simulink model "MRACinSimulink"  (R2025b)
settings: Solver=FixedStepAuto  StartTime=0.0  StopTime=100  FixedStep=0.1  RelTol=1e-3
settings Model: Creator=Asus  LastModifiedBy=Asus

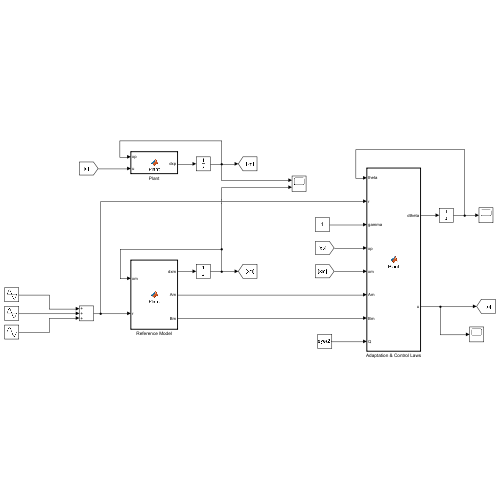
[thumbnail: Simulink's stored preview of the top-level diagram]
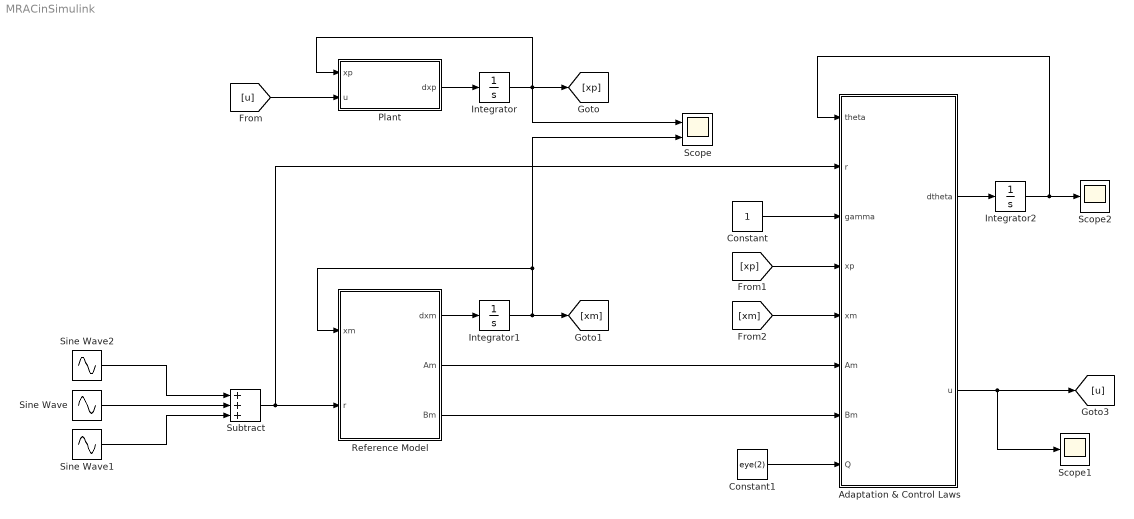
== system MRACinSimulink ==
  Adaptation & Control Laws : MATLAB Function  TreatAsAtomicUnit=on
  Constant : Constant
  Constant1 : Constant  Value=eye(2)
  Integrator : Integrator  InitialCondition=rand(2, 1)
  Integrator1 : Integrator  InitialCondition=rand(2, 1)
  Integrator2 : Integrator  InitialCondition=rand(1, 2)
  Plant : MATLAB Function  TreatAsAtomicUnit=on
  Reference Model : MATLAB Function  TreatAsAtomicUnit=on
  Scope : Scope  NumInputPorts=2
      settings: ActiveDisplayYMinimum=-0.978460666662917  ActiveDisplayYMaximum=1.9226178138046275
  Scope1 : Scope
      settings: ActiveDisplayYMinimum=-10.282022956390476  ActiveDisplayYMaximum=8.9848871674041888
  Scope2 : Scope
      settings: ActiveDisplayYMinimum=-0.32157  ActiveDisplayYMaximum=4.08557  DataLoggingVariableName=ScopeData2
  Sine Wave : Sin  Frequency=2  SampleTime=0
  Sine Wave1 : Sin  Frequency=3  SampleTime=0
  Sine Wave2 : Sin  SampleTime=0
  Subtract : Sum  Inputs=+++
  wires:
  Plant/1(dxp) -> Integrator/1
  Integrator/1 -> Scope/1, [xp], Plant/1(xp)
  Reference Model/1(dxm) -> Integrator1/1
  Integrator1/1 -> [xm], Reference Model/1(xm), Scope/2
  Adaptation & Control Laws/1(dtheta) -> Integrator2/1
  Integrator2/1 -> Scope2/1, Adaptation & Control Laws/1(theta)
  Reference Model/2(Am) -> Adaptation & Control Laws/6(Am)
  Reference Model/3(Bm) -> Adaptation & Control Laws/7(Bm)
  Adaptation & Control Laws/2(u) -> Scope1/1, [u]
  [u] -> Plant/2(u)
  Subtract/1 -> Adaptation & Control Laws/2(r), Reference Model/2(r)
  [xm] -> Adaptation & Control Laws/5(xm)
  [xp] -> Adaptation & Control Laws/4(xp)
  Constant/1 -> Adaptation & Control Laws/3(gamma)
  Constant1/1 -> Adaptation & Control Laws/8(Q)
  Sine Wave2/1 -> Subtract/1
  Sine Wave/1 -> Subtract/2
  Sine Wave1/1 -> Subtract/3

== matlab function MRACinSimulink/Reference Model ==
  data: xm input; dxm output; r input; Am output; Bm output
function [dxm, Am, Bm] = Plant(xm, r)

    Am = [0, 1; -1, -1];
    Bm = [0, 1]';
    
    dxm = Am * xm + Bm * r;

end

== matlab function MRACinSimulink/Plant ==
  data: xp input; dxp output; u input
function dxp = Plant(xp, u)

    Ap = [0, 1; -4, -4];
    Bp = [0, 1]';
    
    dxp = Ap * xp + Bp * u;

end

== matlab function MRACinSimulink/Adaptation & Control Laws ==
  data: theta input; r input; dtheta output; gamma input; xp input; xm input; Am input; Bm input; u output; Q input
function [dtheta, u] = Plant(theta, r, gamma, xp, xm, Am, Bm, Q)
    
    % P      = lyap(Am, Q);
    P = [ 1.5000   -0.5000
         -0.5000    1.0000];
    e      = xp - xm;
    u      = theta' * xp + r;
    dtheta = - gamma * Bm' * P * e * xp';

end
